simulink model "lab3_step9"  (R2019b)
settings: Solver=FixedStepDiscrete  StartTime=0.0  StopTime=stop_time  RelTol=1e-3
InitFcn:
  | sm_callback_init
StopFcn:
  | sm_callback_stop
values from neighbouring files (symbols this model uses):
  delay = 10000    [sm_callback_init.m]
  mp = sm_init_control_signals(mp)    [sm_callback_init.m]    (also in sm_callback_stop.m = sm_stop_verify(mp))
libraries: hdlsllib x10, simulink x3
settings Model: Creator=yassi  LastModifiedBy=asalo
settings DataIOCC: ReturnWorkspaceOutputs=off
settings OptimizationCC: BlockReduction=off  ConditionallyExecuteInputs=off  DefaultParameterBehavior=Inlined
settings DebuggingCC: AlgebraicLoopMsg=error
settings HardwareCC: ProdBitPerPointer=32  ProdBitPerSizeT=32  ProdBitPerPtrDiffT=32  ProdLargestAtomicFloat=None  ProdIntDivRoundTo=Undefined  ProdEndianess=Unspecified  ProdWordSize=32  ProdHWDeviceType=ASIC/FPGA->ASIC/FPGA  TargetBitPerPointer=64  TargetBitPerSizeT=64  TargetBitPerPtrDiffT=64  TargetLongLongMode=on  TargetIntDivRoundTo=Zero  TargetEndianess=LittleEndian  TargetWordSize=64  TargetHWDeviceType=Custom Processor->MATLAB Host Computer  ProdEqTarget=off

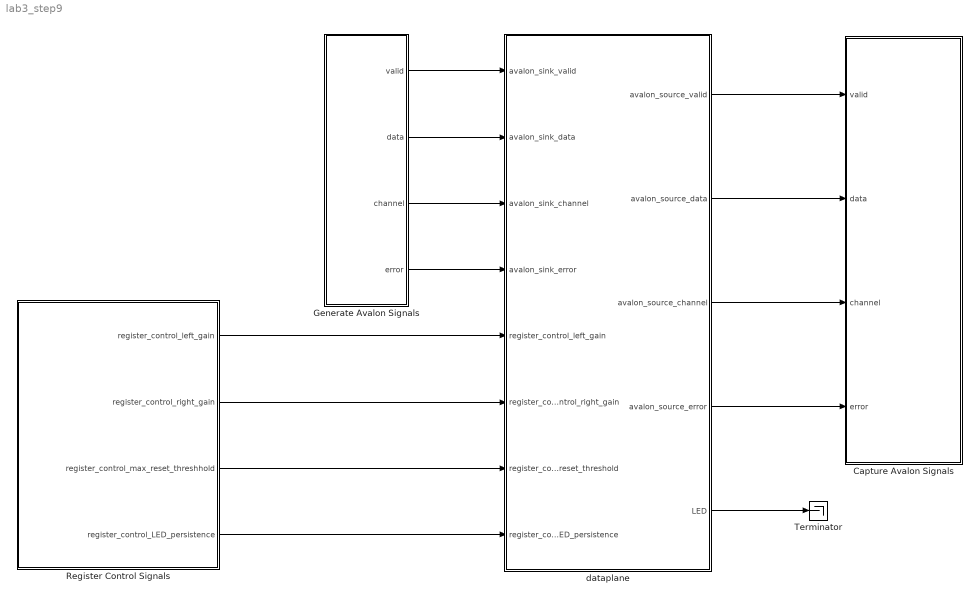
== system lab3_step9 ==
  Capture Avalon Signals : Subsystem
  Generate Avalon Signals : Subsystem
  Register Control Signals : Subsystem
  Terminator : Terminator
  dataplane : Subsystem  TreatAsAtomicUnit=on
  wires:
  Generate Avalon Signals/1(valid) -> dataplane/1(avalon_sink_valid)
  Generate Avalon Signals/2(data) -> dataplane/2(avalon_sink_data)
  Generate Avalon Signals/3(channel) -> dataplane/3(avalon_sink_channel)
  Generate Avalon Signals/4(error) -> dataplane/4(avalon_sink_error)
  dataplane/1(avalon_source_valid) -> Capture Avalon Signals/1(valid)
  dataplane/2(avalon_source_data) -> Capture Avalon Signals/2(data)
  dataplane/3(avalon_source_channel) -> Capture Avalon Signals/3(channel)
  dataplane/4(avalon_source_error) -> Capture Avalon Signals/4(error)
  Register Control Signals/1(register_control_left_gain) -> dataplane/5(register_control_left_gain)
  Register Control Signals/2(register_control_right_gain) -> dataplane/6(register_control_right_gain)
  Register Control Signals/3(register_control_max_reset_threshhold) -> dataplane/7(register_control_max_reset_threshold)
  Register Control Signals/4(register_control_LED_persistence) -> dataplane/8(register_control_LED_persistence)
  dataplane/5(LED) -> Terminator/1

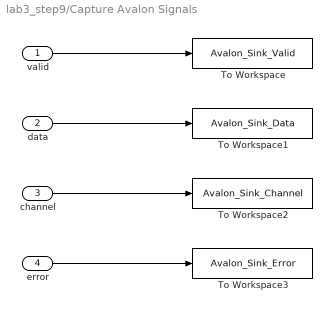
== system lab3_step9/Capture Avalon Signals ==
  valid : Inport
  data : Inport  Port=2
  channel : Inport  Port=3
  error : Inport  Port=4
  To Workspace : ToWorkspace  VariableName=Avalon_Sink_Valid  SaveFormat=Timeseries  SampleTime=-1
  To Workspace1 : ToWorkspace  VariableName=Avalon_Sink_Data  SaveFormat=Timeseries  SampleTime=-1
  To Workspace2 : ToWorkspace  VariableName=Avalon_Sink_Channel  SaveFormat=Timeseries  SampleTime=-1
  To Workspace3 : ToWorkspace  VariableName=Avalon_Sink_Error  SaveFormat=Timeseries  SampleTime=-1
  wires:
  valid/1 -> To Workspace/1
  data/1 -> To Workspace1/1
  channel/1 -> To Workspace2/1
  error/1 -> To Workspace3/1

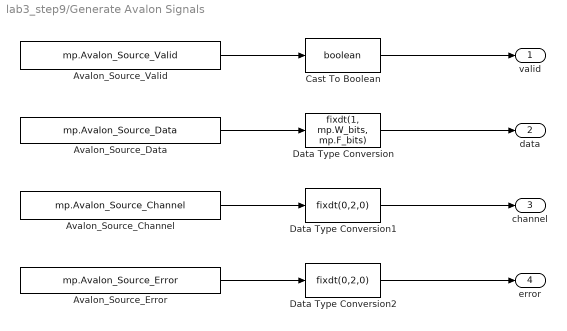
== system lab3_step9/Generate Avalon Signals ==
  Avalon_Source_Channel : FromWorkspace  VariableName=mp.Avalon_Source_Channel  OutDataTypeStr=double  SampleTime=mp.Ts_system
  Avalon_Source_Data : FromWorkspace  VariableName=mp.Avalon_Source_Data  OutDataTypeStr=double  SampleTime=mp.Ts_system
  Avalon_Source_Error : FromWorkspace  VariableName=mp.Avalon_Source_Error  OutDataTypeStr=double  SampleTime=mp.Ts_system
  Avalon_Source_Valid : FromWorkspace  VariableName=mp.Avalon_Source_Valid  OutDataTypeStr=double  SampleTime=mp.Ts_system
  Cast To Boolean : DataTypeConversion  OutDataTypeStr=boolean
  Data Type Conversion : DataTypeConversion  OutDataTypeStr=fixdt(1, mp.W_bits, mp.F_bits)
  Data Type Conversion1 : DataTypeConversion  OutDataTypeStr=fixdt(0,2,0)
  Data Type Conversion2 : DataTypeConversion  OutDataTypeStr=fixdt(0,2,0)
  valid : Outport
  data : Outport  Port=2
  channel : Outport  Port=3
  error : Outport  Port=4
  wires:
  Avalon_Source_Valid/1 -> Cast To Boolean/1
  Avalon_Source_Data/1 -> Data Type Conversion/1
  Avalon_Source_Channel/1 -> Data Type Conversion1/1
  Avalon_Source_Error/1 -> Data Type Conversion2/1
  Cast To Boolean/1 -> valid/1
  Data Type Conversion/1 -> data/1
  Data Type Conversion1/1 -> channel/1
  Data Type Conversion2/1 -> error/1

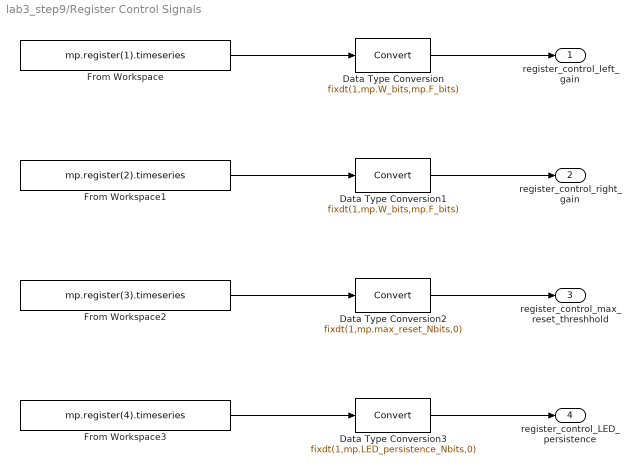
== system lab3_step9/Register Control Signals ==
  Data Type Conversion : DataTypeConversion  OutDataTypeStr=fixdt(1,mp.W_bits,mp.F_bits)
  Data Type Conversion1 : DataTypeConversion  OutDataTypeStr=fixdt(1,mp.W_bits,mp.F_bits)
  Data Type Conversion2 : DataTypeConversion  OutDataTypeStr=fixdt(1,mp.max_reset_Nbits,0)
  Data Type Conversion3 : DataTypeConversion  OutDataTypeStr=fixdt(1,mp.LED_persistence_Nbits,0)
  From Workspace : FromWorkspace  VariableName=mp.register(1).timeseries  OutDataTypeStr=double  SampleTime=mp.Ts_system
  From Workspace1 : FromWorkspace  VariableName=mp.register(2).timeseries  OutDataTypeStr=double  SampleTime=mp.Ts_system
  From Workspace2 : FromWorkspace  VariableName=mp.register(3).timeseries  OutDataTypeStr=double  SampleTime=mp.Ts_system
  From Workspace3 : FromWorkspace  VariableName=mp.register(4).timeseries  OutDataTypeStr=double  SampleTime=mp.Ts_system
  register_control_left_gain : Outport
  register_control_right_gain : Outport  Port=2
  register_control_max_reset_threshhold : Outport  Port=3
  register_control_LED_persistence : Outport  Port=4
  wires:
  Data Type Conversion1/1 -> register_control_right_gain/1
  Data Type Conversion/1 -> register_control_left_gain/1
  From Workspace/1 -> Data Type Conversion/1
  From Workspace1/1 -> Data Type Conversion1/1
  From Workspace2/1 -> Data Type Conversion2/1
  From Workspace3/1 -> Data Type Conversion3/1
  Data Type Conversion3/1 -> register_control_LED_persistence/1
  Data Type Conversion2/1 -> register_control_max_reset_threshhold/1

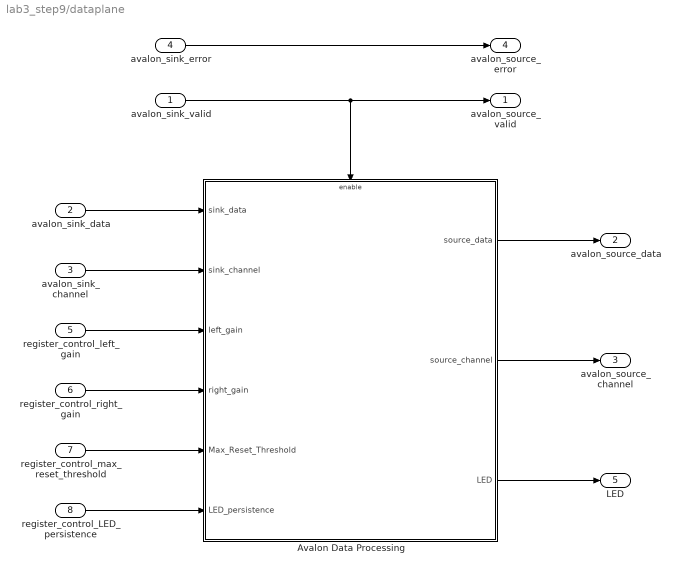
== system lab3_step9/dataplane ==
  avalon_sink_valid : Inport
  avalon_sink_data : Inport  Port=2
  avalon_sink_channel : Inport  Port=3
  avalon_sink_error : Inport  Port=4
  register_control_left_gain : Inport  Port=5
  register_control_right_gain : Inport  Port=6
  register_control_max_reset_threshold : Inport  Port=7
  register_control_LED_persistence : Inport  Port=8
  Avalon Data Processing : Subsystem  TreatAsAtomicUnit=on
  avalon_source_valid : Outport
  avalon_source_data : Outport  Port=2
  avalon_source_channel : Outport  Port=3
  avalon_source_error : Outport  Port=4
  LED : Outport  Port=5
  wires:
  avalon_sink_error/1 -> avalon_source_error/1
  avalon_sink_valid/1 -> avalon_source_valid/1, Avalon Data Processing/Enable
  avalon_sink_data/1 -> Avalon Data Processing/1(sink_data)
  avalon_sink_channel/1 -> Avalon Data Processing/2(sink_channel)
  register_control_left_gain/1 -> Avalon Data Processing/3(left_gain)
  register_control_right_gain/1 -> Avalon Data Processing/4(right_gain)
  Avalon Data Processing/1(source_data) -> avalon_source_data/1
  Avalon Data Processing/2(source_channel) -> avalon_source_channel/1
  Avalon Data Processing/3(LED) -> LED/1
  register_control_max_reset_threshold/1 -> Avalon Data Processing/5(Max_Reset_Threshold)
  register_control_LED_persistence/1 -> Avalon Data Processing/6(LED_persistence)

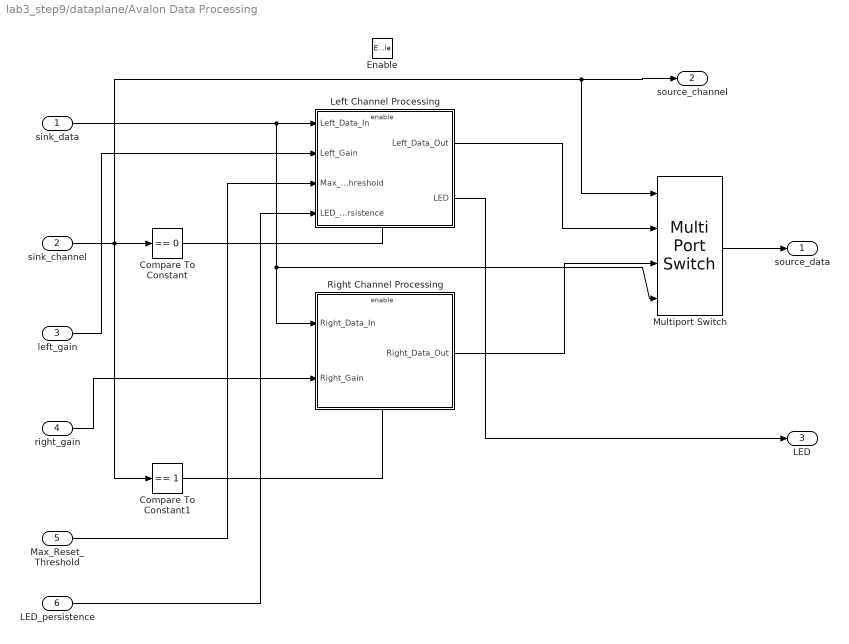
== system lab3_step9/dataplane/Avalon Data Processing ==
  sink_data : Inport
  sink_channel : Inport  Port=2
  left_gain : Inport  Port=3
  right_gain : Inport  Port=4
  Max_Reset_Threshold : Inport  Port=5
  LED_persistence : Inport  Port=6
  Enable : EnablePort
  Compare To Constant : simulink/Logic and Bit Operations/Compare To Constant  relop===  const=0  OutDataTypeStr=boolean
  Compare To Constant1 : simulink/Logic and Bit Operations/Compare To Constant  relop===  const=1  OutDataTypeStr=boolean
  Left Channel Processing : Subsystem  TreatAsAtomicUnit=on
  Multiport Switch : MultiPortSwitch  DataPortOrder=Zero-based contiguous  zeroidx=on
  Right Channel Processing : Subsystem  TreatAsAtomicUnit=on
  source_data : Outport  InitialOutput=0
  source_channel : Outport  Port=2  InitialOutput=0
  LED : Outport  Port=3  InitialOutput=0
  wires:
  sink_data/1 -> Right Channel Processing/1(Right_Data_In), Multiport Switch/4, Left Channel Processing/1(Left_Data_In)
  sink_channel/1 -> source_channel/1, Multiport Switch/1, Compare To Constant1/1, Compare To Constant/1
  Compare To Constant/1 -> Left Channel Processing/Enable
  Compare To Constant1/1 -> Right Channel Processing/Enable
  left_gain/1 -> Left Channel Processing/2(Left_Gain)
  right_gain/1 -> Right Channel Processing/2(Right_Gain)
  Left Channel Processing/1(Left_Data_Out) -> Multiport Switch/2
  Right Channel Processing/1(Right_Data_Out) -> Multiport Switch/3
  Left Channel Processing/2(LED) -> LED/1
  Max_Reset_Threshold/1 -> Left Channel Processing/3(Max_Reset_Threshold)
  LED_persistence/1 -> Left Channel Processing/4(LED_persistence)
  Multiport Switch/1 -> source_data/1

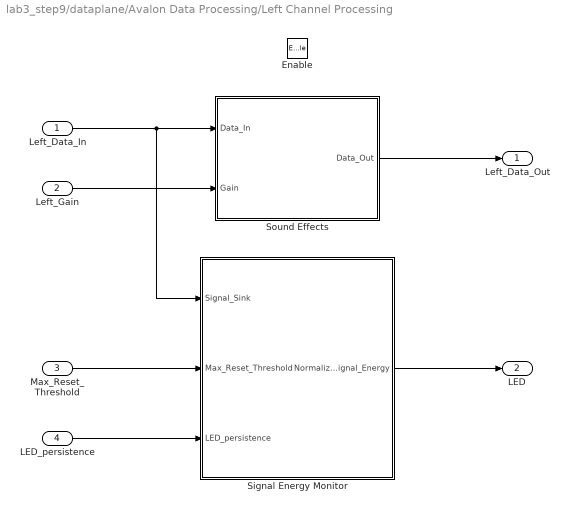
== system lab3_step9/dataplane/Avalon Data Processing/Left Channel Processing ==
  Left_Data_In : Inport
  Left_Gain : Inport  Port=2
  Max_Reset_Threshold : Inport  Port=3
  LED_persistence : Inport  Port=4
  Enable : EnablePort
  Signal Energy Monitor : Subsystem
  Sound Effects : Subsystem
  Left_Data_Out : Outport  InitialOutput=0
  LED : Outport  Port=2  InitialOutput=0
  wires:
  Left_Gain/1 -> Sound Effects/2(Gain)
  Sound Effects/1(Data_Out) -> Left_Data_Out/1
  Left_Data_In/1 -> Signal Energy Monitor/1(Signal_Sink), Sound Effects/1(Data_In)
  Signal Energy Monitor/1(Normalized_Signal_Energy) -> LED/1
  LED_persistence/1 -> Signal Energy Monitor/3(LED_persistence)
  Max_Reset_Threshold/1 -> Signal Energy Monitor/2(Max_Reset_Threshold)

== system lab3_step9/dataplane/Avalon Data Processing/Right Channel Processing ==
  Right_Data_In : Inport
  Right_Gain : Inport  Port=2
  Enable : EnablePort
  Sound Effects : Subsystem
  Right_Data_Out : Outport  InitialOutput=0
  wires:
  Right_Data_In/1 -> Sound Effects/1(Data_In)
  Right_Gain/1 -> Sound Effects/2(Gain)
  Sound Effects/1(Data_Out) -> Right_Data_Out/1

== system lab3_step9/dataplane/Avalon Data Processing/Left Channel Processing/Signal Energy Monitor ==
  Signal_Sink : Inport
  Max_Reset_Threshold : Inport  Port=2
  LED_persistence : Inport  Port=3
  LED_Driver : Subsystem
  Normalize_Signal : Subsystem
  Normalized_Signal_Energy : Outport
  wires:
  Signal_Sink/1 -> Normalize_Signal/1(Signal_Sink)
  Max_Reset_Threshold/1 -> Normalize_Signal/2(Max_Reset_Threshold)
  Normalize_Signal/1(Normalized_Signal_Energy) -> LED_Driver/1(Normalized_Signal)
  LED_Driver/1(LED_Signals) -> Normalized_Signal_Energy/1
  LED_persistence/1 -> LED_Driver/2(LED_persistence)

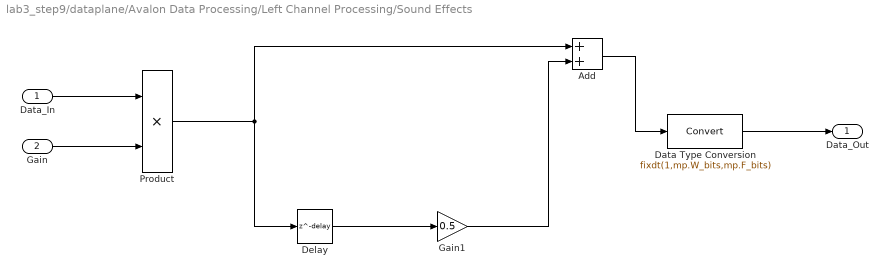
== system lab3_step9/dataplane/Avalon Data Processing/Left Channel Processing/Sound Effects ==
  Data_In : Inport
  Gain : Inport  Port=2
  Add : Sum
  Data Type Conversion : DataTypeConversion  OutDataTypeStr=fixdt(1,mp.W_bits,mp.F_bits)
  Delay : Delay  DelayLength=delay  UseCircularBuffer=on  SampleTime=mp.Ts_system
  Gain1 : Gain  Gain=0.5
  Product : Product
  Data_Out : Outport
  wires:
  Product/1 -> Delay/1, Add/1
  Gain/1 -> Product/2
  Data_In/1 -> Product/1
  Data Type Conversion/1 -> Data_Out/1
  Add/1 -> Data Type Conversion/1
  Delay/1 -> Gain1/1
  Gain1/1 -> Add/2

== system lab3_step9/dataplane/Avalon Data Processing/Right Channel Processing/Sound Effects ==
  Data_In : Inport
  Gain : Inport  Port=2
  Data Type Conversion : DataTypeConversion  OutDataTypeStr=fixdt(1,mp.W_bits,mp.F_bits)
  Product : Product
  Data_Out : Outport
  wires:
  Product/1 -> Data Type Conversion/1
  Data Type Conversion/1 -> Data_Out/1
  Gain/1 -> Product/2
  Data_In/1 -> Product/1

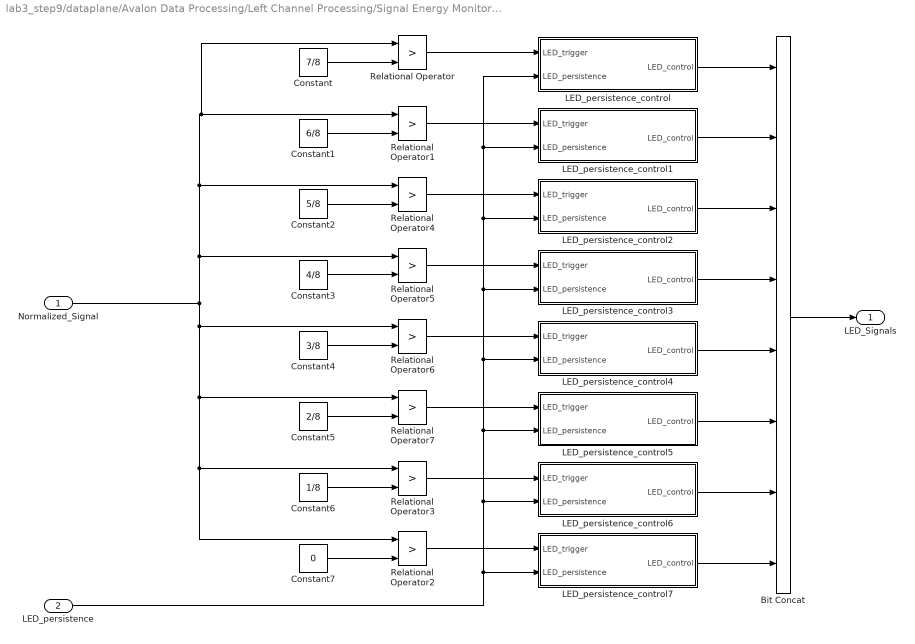
== system lab3_step9/dataplane/Avalon Data Processing/Left Channel Processing/Signal Energy Monitor/LED_Driver ==
  Normalized_Signal : Inport
  LED_persistence : Inport  Port=2
  Bit Concat : hdlsllib/Logic and Bit Operations/Bit Concat  numInputs=8
      settings: SourceProductName=Simulink
  Constant : Constant  Value=7/8  OutDataTypeStr=fixdt(1, mp.W_bits, mp.F_bits)  SampleTime=mp.Ts_system
  Constant1 : Constant  Value=6/8  OutDataTypeStr=fixdt(1, mp.W_bits, mp.F_bits)  SampleTime=mp.Ts_system
  Constant2 : Constant  Value=5/8  OutDataTypeStr=fixdt(1, mp.W_bits, mp.F_bits)  SampleTime=mp.Ts_system
  Constant3 : Constant  Value=4/8  OutDataTypeStr=fixdt(1, mp.W_bits, mp.F_bits)  SampleTime=mp.Ts_system
  Constant4 : Constant  Value=3/8  OutDataTypeStr=fixdt(1, mp.W_bits, mp.F_bits)  SampleTime=mp.Ts_system
  Constant5 : Constant  Value=2/8  OutDataTypeStr=fixdt(1, mp.W_bits, mp.F_bits)  SampleTime=mp.Ts_system
  Constant6 : Constant  Value=1/8  OutDataTypeStr=fixdt(1, mp.W_bits, mp.F_bits)  SampleTime=mp.Ts_system
  Constant7 : Constant  Value=0  OutDataTypeStr=fixdt(1, mp.W_bits, mp.F_bits)  SampleTime=mp.Ts_system
  LED_persistence_control : Subsystem
  LED_persistence_control1 : Subsystem
  LED_persistence_control2 : Subsystem
  LED_persistence_control3 : Subsystem
  LED_persistence_control4 : Subsystem
  LED_persistence_control5 : Subsystem
  LED_persistence_control6 : Subsystem
  LED_persistence_control7 : Subsystem
  Relational Operator{,1..7} (8 alike) : RelationalOperator  Operator=>  OutDataTypeStr=boolean  RndMeth=Simplest
  LED_Signals : Outport
  wires:
  Constant/1 -> Relational Operator/2
  Constant1/1 -> Relational Operator1/2
  Constant2/1 -> Relational Operator4/2
  Constant3/1 -> Relational Operator5/2
  Constant4/1 -> Relational Operator6/2
  Constant5/1 -> Relational Operator7/2
  Constant6/1 -> Relational Operator3/2
  Constant7/1 -> Relational Operator2/2
  Normalized_Signal/1 -> Relational Operator6/1, Relational Operator7/1, Relational Operator3/1, Relational Operator2/1, Relational Operator5/1, Relational Operator4/1, Relational Operator/1, Relational Operator1/1
  Bit Concat/1 -> LED_Signals/1
  Relational Operator/1 -> LED_persistence_control/1(LED_trigger)
  Relational Operator1/1 -> LED_persistence_control1/1(LED_trigger)
  Relational Operator5/1 -> LED_persistence_control3/1(LED_trigger)
  Relational Operator4/1 -> LED_persistence_control2/1(LED_trigger)
  Relational Operator7/1 -> LED_persistence_control5/1(LED_trigger)
  Relational Operator2/1 -> LED_persistence_control7/1(LED_trigger)
  Relational Operator3/1 -> LED_persistence_control6/1(LED_trigger)
  Relational Operator6/1 -> LED_persistence_control4/1(LED_trigger)
  LED_persistence/1 -> LED_persistence_control7/2(LED_persistence), LED_persistence_control6/2(LED_persistence), LED_persistence_control5/2(LED_persistence), LED_persistence_control4/2(LED_persistence), LED_persistence_control3/2(LED_persistence), LED_persistence_control2/2(LED_persistence), LED_persistence_control1/2(LED_persistence), LED_persistence_control/2(LED_persistence)
  LED_persistence_control1/1(LED_control) -> Bit Concat/2
  LED_persistence_control/1(LED_control) -> Bit Concat/1
  LED_persistence_control2/1(LED_control) -> Bit Concat/3
  LED_persistence_control3/1(LED_control) -> Bit Concat/4
  LED_persistence_control4/1(LED_control) -> Bit Concat/5
  LED_persistence_control5/1(LED_control) -> Bit Concat/6
  LED_persistence_control6/1(LED_control) -> Bit Concat/7
  LED_persistence_control7/1(LED_control) -> Bit Concat/8

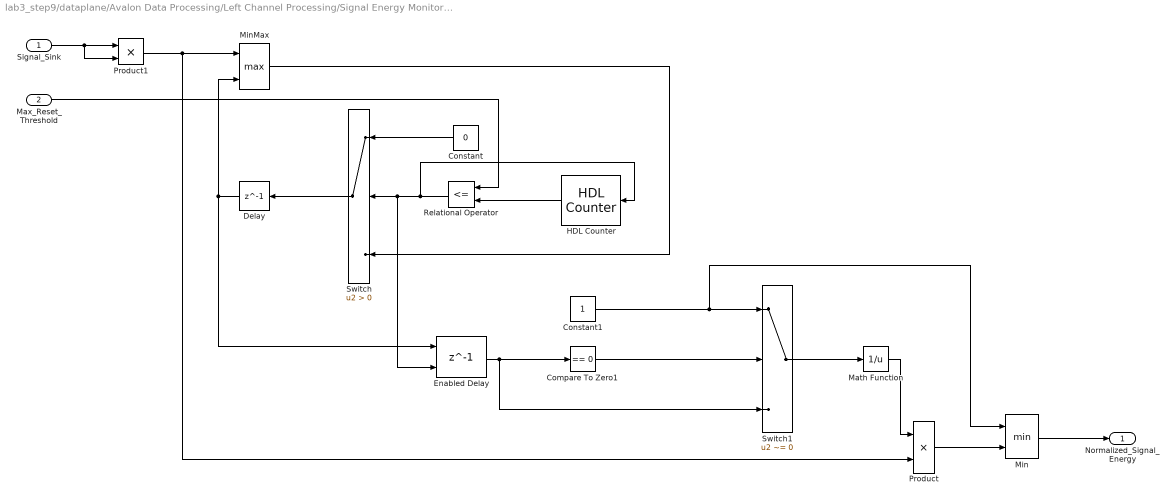
== system lab3_step9/dataplane/Avalon Data Processing/Left Channel Processing/Signal Energy Monitor/Normalize_Signal ==
  Signal_Sink : Inport
  Max_Reset_Threshold : Inport  Port=2
  Compare To Zero1 : simulink/Logic and Bit Operations/Compare To Zero  relop===  OutDataTypeStr=boolean
  Constant : Constant  Value=0  OutDataTypeStr=fixdt(1,mp.W_bits,mp.F_bits)  SampleTime=mp.Ts_system
  Constant1 : Constant  OutDataTypeStr=fixdt(1,mp.W_bits,mp.F_bits)  SampleTime=mp.Ts_system
  Delay : Delay  DelayLength=1
  Enabled Delay : Delay  DelayLength=1  ShowEnablePort=on
      settings: InputPortMap=u0,e6
  HDL Counter : hdlsllib/Sources/HDL Counter  CountType=Free running  CountInit=0  CountStep=1  CountMax=25  CountFromType=Initial value  CountFrom=0  CountResetPort=on  CountLoadPort=off  CountEnbPort=off  CountDirPort=off  CountDataType=Unsigned  CountWordLen=mp.max_reset_Nbits  CountFracLen=0  CountSampTime=1
      settings: SourceProductName=Simulink
  Math Function : Math  Operator=reciprocal  SignedPower=off  OutDataTypeStr=fixdt(1,32,24)  RndMeth=Zero  SaturateOnIntegerOverflow=on
  Min : MinMax  Inputs=2
  MinMax : MinMax  Function=max  Inputs=2
  Product : Product  OutDataTypeStr=fixdt(1,32,28)
  Product1 : Product  OutDataTypeStr=fixdt(1,mp.W_bits,mp.F_bits)
  Relational Operator : RelationalOperator  Operator=<=  OutDataTypeStr=boolean  RndMeth=Nearest
  Switch : Switch  Criteria=u2 > Threshold
  Switch1 : Switch  Criteria=u2 ~= 0
  Normalized_Signal_Energy : Outport
  wires:
  Delay/1 -> Enabled Delay/1, MinMax/2
  Enabled Delay/1 -> Switch1/3, Compare To Zero1/1
  MinMax/1 -> Switch/3
  Relational Operator/1 -> HDL Counter/1, Enabled Delay/2, Switch/2
  Compare To Zero1/1 -> Switch1/2
  HDL Counter/1 -> Relational Operator/2
  Product/1 -> Min/2
  Product1/1 -> Product/2, MinMax/1
  Math Function/1 -> Product/1
  Constant1/1 -> Min/1, Switch1/1
  Constant/1 -> Switch/1
  Switch/1 -> Delay/1
  Min/1 -> Normalized_Signal_Energy/1
  Switch1/1 -> Math Function/1
  Signal_Sink/1 -> Product1/2, Product1/1
  Max_Reset_Threshold/1 -> Relational Operator/1

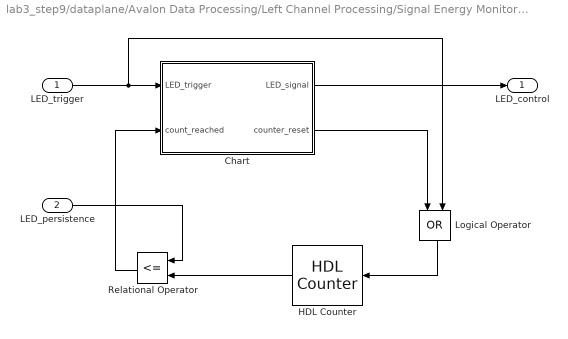
== system lab3_step9/dataplane/Avalon Data Processing/Left Channel Processing/Signal Energy Monitor/LED_Driver/LED_persistence_control ==
  LED_trigger : Inport
  LED_persistence : Inport  Port=2
  Chart : Stateflow chart  BlockKeywords=__PRM__SERIALIZED__DATA__:Stateflow Chart,Stateflow Diagram  TreatAsAtomicUnit=on
  HDL Counter : hdlsllib/Sources/HDL Counter  CountType=Free running  CountInit=0  CountStep=1  CountMax=25  CountFromType=Initial value  CountFrom=0  CountResetPort=on  CountLoadPort=off  CountEnbPort=off  CountDirPort=off  CountDataType=Unsigned  CountWordLen=mp.LED_persistence_Nbits  CountFracLen=0  CountSampTime=1
      settings: SourceProductName=Simulink
  Logical Operator : Logic  Operator=OR  AllPortsSameDT=off  OutDataTypeStr=boolean
  Relational Operator : RelationalOperator  Operator=<=  OutDataTypeStr=boolean  RndMeth=Simplest
  LED_control : Outport
  wires:
  LED_trigger/1 -> Logical Operator/2, Chart/1(LED_trigger)
  Chart/2(counter_reset) -> Logical Operator/1
  Logical Operator/1 -> HDL Counter/1
  HDL Counter/1 -> Relational Operator/2
  LED_persistence/1 -> Relational Operator/1
  Relational Operator/1 -> Chart/2(count_reached)
  Chart/1(LED_signal) -> LED_control/1

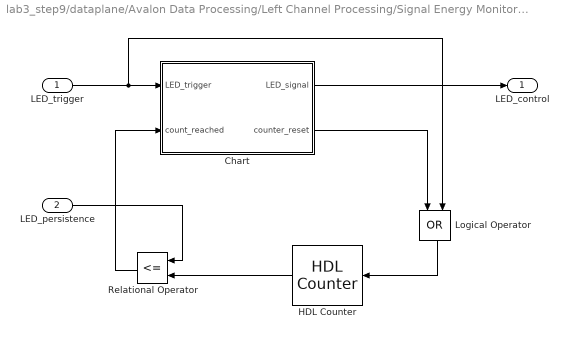
== system lab3_step9/dataplane/Avalon Data Processing/Left Channel Processing/Signal Energy Monitor/LED_Driver/LED_persistence_control1 ==
  LED_trigger : Inport
  LED_persistence : Inport  Port=2
  Chart : Stateflow chart  BlockKeywords=__PRM__SERIALIZED__DATA__:Stateflow Chart,Stateflow Diagram  TreatAsAtomicUnit=on
  HDL Counter : hdlsllib/Sources/HDL Counter  CountType=Count limited  CountInit=0  CountStep=1  CountMax=25  CountFromType=Initial value  CountFrom=0  CountResetPort=on  CountLoadPort=off  CountEnbPort=off  CountDirPort=off  CountDataType=Unsigned  CountWordLen=mp.LED_persistence_Nbits  CountFracLen=0  CountSampTime=1
      settings: SourceProductName=Simulink
  Logical Operator : Logic  Operator=OR  AllPortsSameDT=off  OutDataTypeStr=boolean
  Relational Operator : RelationalOperator  Operator=<=  OutDataTypeStr=boolean  RndMeth=Simplest
  LED_control : Outport
  wires:
  LED_trigger/1 -> Logical Operator/2, Chart/1(LED_trigger)
  Chart/2(counter_reset) -> Logical Operator/1
  Logical Operator/1 -> HDL Counter/1
  HDL Counter/1 -> Relational Operator/2
  LED_persistence/1 -> Relational Operator/1
  Relational Operator/1 -> Chart/2(count_reached)
  Chart/1(LED_signal) -> LED_control/1

== system lab3_step9/dataplane/Avalon Data Processing/Left Channel Processing/Signal Energy Monitor/LED_Driver/LED_persistence_control2 ==
  LED_trigger : Inport
  LED_persistence : Inport  Port=2
  Chart : Stateflow chart  BlockKeywords=__PRM__SERIALIZED__DATA__:Stateflow Chart,Stateflow Diagram  TreatAsAtomicUnit=on
  HDL Counter : hdlsllib/Sources/HDL Counter  CountType=Count limited  CountInit=0  CountStep=1  CountMax=25  CountFromType=Initial value  CountFrom=0  CountResetPort=on  CountLoadPort=off  CountEnbPort=off  CountDirPort=off  CountDataType=Unsigned  CountWordLen=mp.LED_persistence_Nbits  CountFracLen=0  CountSampTime=1
      settings: SourceProductName=Simulink
  Logical Operator : Logic  Operator=OR  AllPortsSameDT=off  OutDataTypeStr=boolean
  Relational Operator : RelationalOperator  Operator=<=  OutDataTypeStr=boolean  RndMeth=Simplest
  LED_control : Outport
  wires:
  LED_trigger/1 -> Logical Operator/2, Chart/1(LED_trigger)
  Chart/2(counter_reset) -> Logical Operator/1
  Logical Operator/1 -> HDL Counter/1
  HDL Counter/1 -> Relational Operator/2
  LED_persistence/1 -> Relational Operator/1
  Relational Operator/1 -> Chart/2(count_reached)
  Chart/1(LED_signal) -> LED_control/1

== system lab3_step9/dataplane/Avalon Data Processing/Left Channel Processing/Signal Energy Monitor/LED_Driver/LED_persistence_control3 ==
  LED_trigger : Inport
  LED_persistence : Inport  Port=2
  Chart : Stateflow chart  BlockKeywords=__PRM__SERIALIZED__DATA__:Stateflow Chart,Stateflow Diagram  TreatAsAtomicUnit=on
  HDL Counter : hdlsllib/Sources/HDL Counter  CountType=Count limited  CountInit=0  CountStep=1  CountMax=25  CountFromType=Initial value  CountFrom=0  CountResetPort=on  CountLoadPort=off  CountEnbPort=off  CountDirPort=off  CountDataType=Unsigned  CountWordLen=mp.LED_persistence_Nbits  CountFracLen=0  CountSampTime=1
      settings: SourceProductName=Simulink
  Logical Operator : Logic  Operator=OR  AllPortsSameDT=off  OutDataTypeStr=boolean
  Relational Operator : RelationalOperator  Operator=<=  OutDataTypeStr=boolean  RndMeth=Simplest
  LED_control : Outport
  wires:
  LED_trigger/1 -> Logical Operator/2, Chart/1(LED_trigger)
  Chart/2(counter_reset) -> Logical Operator/1
  Logical Operator/1 -> HDL Counter/1
  HDL Counter/1 -> Relational Operator/2
  LED_persistence/1 -> Relational Operator/1
  Relational Operator/1 -> Chart/2(count_reached)
  Chart/1(LED_signal) -> LED_control/1

== system lab3_step9/dataplane/Avalon Data Processing/Left Channel Processing/Signal Energy Monitor/LED_Driver/LED_persistence_control4 ==
  LED_trigger : Inport
  LED_persistence : Inport  Port=2
  Chart : Stateflow chart  BlockKeywords=__PRM__SERIALIZED__DATA__:Stateflow Chart,Stateflow Diagram  TreatAsAtomicUnit=on
  HDL Counter : hdlsllib/Sources/HDL Counter  CountType=Count limited  CountInit=0  CountStep=1  CountMax=25  CountFromType=Initial value  CountFrom=0  CountResetPort=on  CountLoadPort=off  CountEnbPort=off  CountDirPort=off  CountDataType=Unsigned  CountWordLen=mp.LED_persistence_Nbits  CountFracLen=0  CountSampTime=1
      settings: SourceProductName=Simulink
  Logical Operator : Logic  Operator=OR  AllPortsSameDT=off  OutDataTypeStr=boolean
  Relational Operator : RelationalOperator  Operator=<=  OutDataTypeStr=boolean  RndMeth=Simplest
  LED_control : Outport
  wires:
  LED_trigger/1 -> Logical Operator/2, Chart/1(LED_trigger)
  Chart/2(counter_reset) -> Logical Operator/1
  Logical Operator/1 -> HDL Counter/1
  HDL Counter/1 -> Relational Operator/2
  LED_persistence/1 -> Relational Operator/1
  Relational Operator/1 -> Chart/2(count_reached)
  Chart/1(LED_signal) -> LED_control/1

== system lab3_step9/dataplane/Avalon Data Processing/Left Channel Processing/Signal Energy Monitor/LED_Driver/LED_persistence_control5 ==
  LED_trigger : Inport
  LED_persistence : Inport  Port=2
  Chart : Stateflow chart  BlockKeywords=__PRM__SERIALIZED__DATA__:Stateflow Chart,Stateflow Diagram  TreatAsAtomicUnit=on
  HDL Counter : hdlsllib/Sources/HDL Counter  CountType=Count limited  CountInit=0  CountStep=1  CountMax=25  CountFromType=Initial value  CountFrom=0  CountResetPort=on  CountLoadPort=off  CountEnbPort=off  CountDirPort=off  CountDataType=Unsigned  CountWordLen=mp.LED_persistence_Nbits  CountFracLen=0  CountSampTime=1
      settings: SourceProductName=Simulink
  Logical Operator : Logic  Operator=OR  AllPortsSameDT=off  OutDataTypeStr=boolean
  Relational Operator : RelationalOperator  Operator=<=  OutDataTypeStr=boolean  RndMeth=Simplest
  LED_control : Outport
  wires:
  LED_trigger/1 -> Logical Operator/2, Chart/1(LED_trigger)
  Chart/2(counter_reset) -> Logical Operator/1
  Logical Operator/1 -> HDL Counter/1
  HDL Counter/1 -> Relational Operator/2
  LED_persistence/1 -> Relational Operator/1
  Relational Operator/1 -> Chart/2(count_reached)
  Chart/1(LED_signal) -> LED_control/1

== system lab3_step9/dataplane/Avalon Data Processing/Left Channel Processing/Signal Energy Monitor/LED_Driver/LED_persistence_control6 ==
  LED_trigger : Inport
  LED_persistence : Inport  Port=2
  Chart : Stateflow chart  BlockKeywords=__PRM__SERIALIZED__DATA__:Stateflow Chart,Stateflow Diagram  TreatAsAtomicUnit=on
  HDL Counter : hdlsllib/Sources/HDL Counter  CountType=Count limited  CountInit=0  CountStep=1  CountMax=25  CountFromType=Initial value  CountFrom=0  CountResetPort=on  CountLoadPort=off  CountEnbPort=off  CountDirPort=off  CountDataType=Unsigned  CountWordLen=mp.LED_persistence_Nbits  CountFracLen=0  CountSampTime=1
      settings: SourceProductName=Simulink
  Logical Operator : Logic  Operator=OR  AllPortsSameDT=off  OutDataTypeStr=boolean
  Relational Operator : RelationalOperator  Operator=<=  OutDataTypeStr=boolean  RndMeth=Simplest
  LED_control : Outport
  wires:
  LED_trigger/1 -> Logical Operator/2, Chart/1(LED_trigger)
  Chart/2(counter_reset) -> Logical Operator/1
  Logical Operator/1 -> HDL Counter/1
  HDL Counter/1 -> Relational Operator/2
  LED_persistence/1 -> Relational Operator/1
  Relational Operator/1 -> Chart/2(count_reached)
  Chart/1(LED_signal) -> LED_control/1

== system lab3_step9/dataplane/Avalon Data Processing/Left Channel Processing/Signal Energy Monitor/LED_Driver/LED_persistence_control7 ==
  LED_trigger : Inport
  LED_persistence : Inport  Port=2
  Chart : Stateflow chart  BlockKeywords=__PRM__SERIALIZED__DATA__:Stateflow Chart,Stateflow Diagram  TreatAsAtomicUnit=on
  HDL Counter : hdlsllib/Sources/HDL Counter  CountType=Count limited  CountInit=0  CountStep=1  CountMax=25  CountFromType=Initial value  CountFrom=0  CountResetPort=on  CountLoadPort=off  CountEnbPort=off  CountDirPort=off  CountDataType=Unsigned  CountWordLen=mp.LED_persistence_Nbits  CountFracLen=0  CountSampTime=1
      settings: SourceProductName=Simulink
  Logical Operator : Logic  Operator=OR  AllPortsSameDT=off  OutDataTypeStr=boolean
  Relational Operator : RelationalOperator  Operator=<=  OutDataTypeStr=boolean  RndMeth=Simplest
  LED_control : Outport
  wires:
  LED_trigger/1 -> Logical Operator/2, Chart/1(LED_trigger)
  Chart/2(counter_reset) -> Logical Operator/1
  Logical Operator/1 -> HDL Counter/1
  HDL Counter/1 -> Relational Operator/2
  LED_persistence/1 -> Relational Operator/1
  Relational Operator/1 -> Chart/2(count_reached)
  Chart/1(LED_signal) -> LED_control/1

== stateflow chart lab3_step9/dataplane/Avalon Data Processing/Left Channel Processing/Signal Energy Monitor/LED_Driver/LED_persistence_control1/Chart ==
  settings: executeAtInitialization=1
  state LED_off
    entry: LED_signal=false;
    entry: counter_reset=true;
  state LED_on
    entry: LED_signal=true;
    entry: counter_reset=false;
  (default) -> LED_off
  LED_off -> LED_on : [LED_trigger==1]
  LED_on -> LED_off : [count_reached==1]
  data: LED_trigger input; count_reached input; LED_signal output; counter_reset output

== stateflow chart lab3_step9/dataplane/Avalon Data Processing/Left Channel Processing/Signal Energy Monitor/LED_Driver/LED_persistence_control/Chart ==
  settings: executeAtInitialization=1
  state LED_off
    entry: LED_signal=false;
    entry: counter_reset=true;
  state LED_on
    entry: LED_signal=true;
    entry: counter_reset=false;
  (default) -> LED_off
  LED_off -> LED_on : [LED_trigger==1]
  LED_on -> LED_off : [count_reached==1]
  data: LED_trigger input; count_reached input; LED_signal output; counter_reset output

== stateflow chart lab3_step9/dataplane/Avalon Data Processing/Left Channel Processing/Signal Energy Monitor/LED_Driver/LED_persistence_control2/Chart ==
  settings: executeAtInitialization=1
  state LED_off
    entry: LED_signal=false;
    entry: counter_reset=true;
  state LED_on
    entry: LED_signal=true;
    entry: counter_reset=false;
  (default) -> LED_off
  LED_off -> LED_on : [LED_trigger==1]
  LED_on -> LED_off : [count_reached==1]
  data: LED_trigger input; count_reached input; LED_signal output; counter_reset output

== stateflow chart lab3_step9/dataplane/Avalon Data Processing/Left Channel Processing/Signal Energy Monitor/LED_Driver/LED_persistence_control3/Chart ==
  settings: executeAtInitialization=1
  state LED_off
    entry: LED_signal=false;
    entry: counter_reset=true;
  state LED_on
    entry: LED_signal=true;
    entry: counter_reset=false;
  (default) -> LED_off
  LED_off -> LED_on : [LED_trigger==1]
  LED_on -> LED_off : [count_reached==1]
  data: LED_trigger input; count_reached input; LED_signal output; counter_reset output

== stateflow chart lab3_step9/dataplane/Avalon Data Processing/Left Channel Processing/Signal Energy Monitor/LED_Driver/LED_persistence_control4/Chart ==
  settings: executeAtInitialization=1
  state LED_off
    entry: LED_signal=false;
    entry: counter_reset=true;
  state LED_on
    entry: LED_signal=true;
    entry: counter_reset=false;
  (default) -> LED_off
  LED_off -> LED_on : [LED_trigger==1]
  LED_on -> LED_off : [count_reached==1]
  data: LED_trigger input; count_reached input; LED_signal output; counter_reset output

== stateflow chart lab3_step9/dataplane/Avalon Data Processing/Left Channel Processing/Signal Energy Monitor/LED_Driver/LED_persistence_control5/Chart ==
  settings: executeAtInitialization=1
  state LED_off
    entry: LED_signal=false;
    entry: counter_reset=true;
  state LED_on
    entry: LED_signal=true;
    entry: counter_reset=false;
  (default) -> LED_off
  LED_off -> LED_on : [LED_trigger==1]
  LED_on -> LED_off : [count_reached==1]
  data: LED_trigger input; count_reached input; LED_signal output; counter_reset output

== stateflow chart lab3_step9/dataplane/Avalon Data Processing/Left Channel Processing/Signal Energy Monitor/LED_Driver/LED_persistence_control6/Chart ==
  settings: executeAtInitialization=1
  state LED_off
    entry: LED_signal=false;
    entry: counter_reset=true;
  state LED_on
    entry: LED_signal=true;
    entry: counter_reset=false;
  (default) -> LED_off
  LED_off -> LED_on : [LED_trigger==1]
  LED_on -> LED_off : [count_reached==1]
  data: LED_trigger input; count_reached input; LED_signal output; counter_reset output

== stateflow chart lab3_step9/dataplane/Avalon Data Processing/Left Channel Processing/Signal Energy Monitor/LED_Driver/LED_persistence_control7/Chart ==
  settings: executeAtInitialization=1
  state LED_off
    entry: LED_signal=false;
    entry: counter_reset=true;
  state LED_on
    entry: LED_signal=true;
    entry: counter_reset=false;
  (default) -> LED_off
  LED_off -> LED_on : [LED_trigger==1]
  LED_on -> LED_off : [count_reached==1]
  data: LED_trigger input; count_reached input; LED_signal output; counter_reset output
